simulink model "Pendule_Observateur_Controleur_Continu"  (R2014b)
settings: Solver=ode45  StartTime=0.0  StopTime=10.0  RelTol=1e-3
values from neighbouring files (symbols this model uses):
  A = zeros (4,4)    [Modele_Pendule.m]
  Ao = A-Ko*C    [Design_Matlab_File_Pendule_IMC_.m]
  B = zeros (4,1)    [Modele_Pendule.m]
  Bo = [B Ko]    [Design_Matlab_File_Pendule_IMC_.m]
  C = [1 0 0 0 ... (first row only)    [Modele_Pendule.m]
  Co = eye(4,4)    [Design_Matlab_File_Pendule_IMC_.m]
  D = [ 0 0 ]'    [Modele_Pendule.m]
  Do = zeros(4,3)    [Design_Matlab_File_Pendule_IMC_.m]
  Kc = place (A,B,Pc)    [Design_Matlab_File_Pendule_IMC_.m]
  X0_o = [0 0 0 0]'    [Design_Matlab_File_Pendule_IMC_.m]
libraries: simulink_extras x1
settings Model: Creator=ArbenCela  LastModifiedBy=ArbenCela

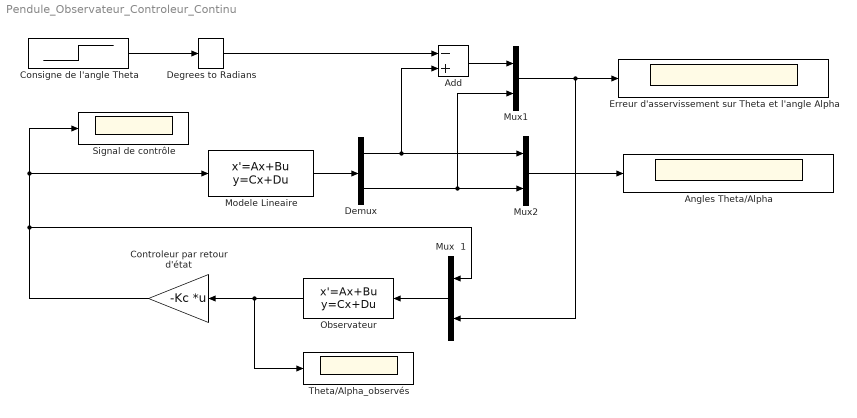
== system Pendule_Observateur_Controleur_Continu ==
  Add : Sum  Inputs=-+
  Angles Theta/Alpha : Scope
  Consigne de l'angle Theta : Step  Time=6  After=50  SampleTime=0
  "Controleur par retour d'état " : Gain  Gain=-Kc  Multiplication=Matrix(K*u)  SaturateOnIntegerOverflow=on  OutDataTypeStr=Inherit: Same as input  ParamDataTypeStr=Inherit: Same as input
  Degrees to Radians : simulink_extras/Transformations/Degrees to Radians
  Demux : Demux  Outputs=2
  Erreur d'asservissement sur Theta et l'angle Alpha : Scope
      settings: SaveName=ScopeData2
  Modele Lineaire : StateSpace  A=A  B=B  C=C  D=D  X0=[0.2,0.2,0,0]
  Mux  1 : Mux  Inputs=2
  Mux1 : Mux  Inputs=2
  Mux2 : Mux  Inputs=2
  Observateur : StateSpace  A=Ao  B=Bo  C=Co  D=Do  X0=X0_o
  "Signal de contrôle " : Scope
      settings: SaveName=ScopeData3
  Theta/Alpha_observés : Scope
  wires:
  "Controleur par retour d'état "/1 -> Mux  1/1, Modele Lineaire/1, "Signal de contrôle "/1
  Observateur/1 -> Theta/Alpha_observés/1, "Controleur par retour d'état "/1
  Mux  1/1 -> Observateur/1
  Consigne de l'angle Theta/1 -> Degrees to Radians/1
  Degrees to Radians/1 -> Add/1
  Add/1 -> Mux1/1
  Modele Lineaire/1 -> Demux/1
  Demux/1 -> Add/2, Mux2/1
  Demux/2 -> Mux1/2, Mux2/2
  Mux1/1 -> Mux  1/2, Erreur d'asservissement sur Theta et l'angle Alpha/1
  Mux2/1 -> Angles Theta/Alpha/1
